simulink model "gm_TWO_BIT_ADDER"  (R2022b)
settings: Solver=FixedStepDiscrete  StartTime=0.0  StopTime=10.0  RelTol=1e-3
settings Model: Creator=saran  LastModifiedBy=saran
settings SolverCC: AlgebraicLoopSolver=TrustRegion  AutoInsertRateTranBlk=on
settings DataIOCC: LimitDataPoints=on  SaveOutput=off  SaveTime=off
settings OptimizationCC: BlockReduction=off  ConditionallyExecuteInputs=off  DefaultParameterBehavior=Inlined  LifeSpan=inf
settings DebuggingCC: AlgebraicLoopMsg=error  InheritedTsInSrcMsg=none  SingleTaskRateTransMsg=error  UnconnectedInputMsg=warning  UnconnectedOutputMsg=warning  UnconnectedLineMsg=warning  AllowSymbolicDim=off  StrictBusMsg=ErrorOnBusTreatedAsVector  SFUnexpectedBacktrackingDiag=warning  SFNoUnconditionalDefaultTransitionDiag=warning  SFExecutionAtInitializationDiag=none  SFMachineParentedDataDiag=warning  ArithmeticOperatorsInVariantConditions=warning
settings HardwareCC: ProdBitPerPointer=32  ProdBitPerSizeT=32  ProdBitPerPtrDiffT=32  ProdLargestAtomicFloat=None  ProdIntDivRoundTo=Undefined  ProdEndianess=Unspecified  ProdWordSize=32  ProdHWDeviceType=ASIC/FPGA->ASIC/FPGA  ProdEqTarget=off
settings ModelReferenceCC: EnableRefExpFcnMdlSchedulingChecks=on
settings SFSimCC: SimUseLocalCustomCode=off  CustomCodeUndefinedFunction=UseInterfaceOnly
settings RTWCC: RTWUseLocalCustomCode=off
settings CodeAppCC: StateflowObjectComments=on
settings GRTTargetCC: TargetLangStandard=C89/C90 (ANSI)
settings ConfigComp: CovScope=ReferencedModels  CovMetricSettings=dw  CovSaveCumulativeToWorkspaceVar=on  CovSaveSingleToWorkspaceVar=on  CovExternalEMLEnable=off  CovSFcnEnable=off

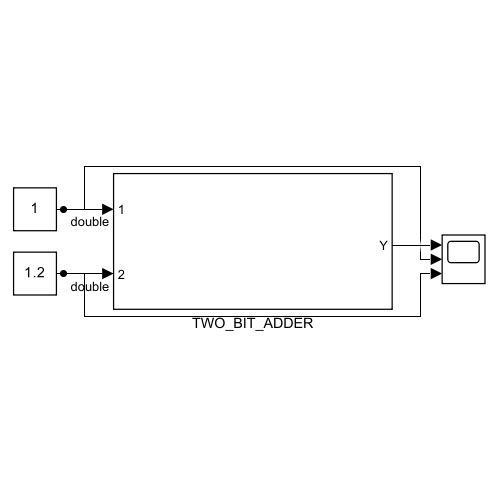
[thumbnail: Simulink's stored preview of the top-level diagram]
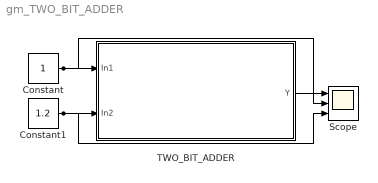
== system gm_TWO_BIT_ADDER ==
  Constant : Constant  SampleTime=1
  Constant1 : Constant  Value=1.2  SampleTime=1
  Scope : Scope  NumInputPorts=3
  TWO_BIT_ADDER : Subsystem
  wires:
  Constant1/1 -> TWO_BIT_ADDER/2(In2), Scope/3
  Constant/1 -> TWO_BIT_ADDER/1(In1), Scope/2
  TWO_BIT_ADDER/1(Y) -> Scope/1

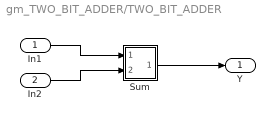
== system gm_TWO_BIT_ADDER/TWO_BIT_ADDER ==
  In1 : Inport  OutDataTypeStr=double  PortDimensions=1  SampleTime=1
  In2 : Inport  Port=2  OutDataTypeStr=double  PortDimensions=1  SampleTime=1
  Sum : Subsystem
      mask Display: disp('NFP\nadd');
  Y : Outport  SampleTime=1  VectorParamsAs1DForOutWhenUnconnected=off
  wires:
  In1/1 -> Sum/1(In1)
  In2/1 -> Sum/2(In2)
  Sum/1(Out1) -> Y/1

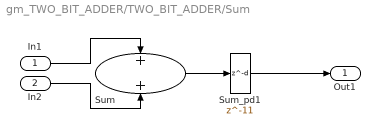
== system gm_TWO_BIT_ADDER/TWO_BIT_ADDER/Sum ==
  In1 : Inport
  In2 : Inport  Port=2
  Sum : Sum  OutDataTypeStr=double  SampleTime=1
  Sum_pd1 : Delay  DelayLength=11
  Out1 : Outport
  wires:
  In1/1 -> Sum/1
  In2/1 -> Sum/2
  Sum/1 -> Sum_pd1/1
  Sum_pd1/1 -> Out1/1
